simulink model "controller_pid_sim_model_exp_comp"  (R2014b)
settings: Solver=ode45  StartTime=0.0  StopTime=10.0  RelTol=1e-3
values from neighbouring files (symbols this model uses):
  Dr_phi = 0.12*100    (= 12)    [defineGains.m]    (also in gain_tuning.m; model_exp_comparison.m)
  Dr_theta = 0.12*100    (= 12)    [defineGains.m]    (also in gain_tuning.m; model_exp_comparison.m)
  Dvx = 0    [defineGains.m]    (also in gain_tuning.m; model_exp_comparison.m)
  Dvy = 0    [defineGains.m]    (also in gain_tuning.m; model_exp_comparison.m)
  Dx = 0    [defineGains.m]    (also in gain_tuning.m; model_exp_comparison.m)
  Dy = 0    [defineGains.m]    (also in gain_tuning.m; model_exp_comparison.m)
  g = 9.81    [gain_tuning.m]    (also in gain_tuning_noise.m; model_exp_comparison.m; transfer_functions.m)
  Ir_phi = -0.005*100    (= -0.5)    [defineGains.m]    (also in gain_tuning.m; model_exp_comparison.m)
  Ir_theta = -0.005*100    (= -0.5)    [defineGains.m]    (also in gain_tuning.m; model_exp_comparison.m)
  Ivx = -0.05    [defineGains.m]    (also in gain_tuning.m; model_exp_comparison.m)
  Ivy = 0.05    [defineGains.m]    (also in gain_tuning.m; model_exp_comparison.m)
  Ix = 0    [defineGains.m]    (also in gain_tuning.m; model_exp_comparison.m = 0.02)
  Iy = 0    [defineGains.m]    (also in gain_tuning.m; model_exp_comparison.m = 0.03)
  Pa_phi = 10    [defineGains.m]    (also in gain_tuning.m; model_exp_comparison.m)
  Pa_theta = 10    [defineGains.m]    (also in gain_tuning.m; model_exp_comparison.m)
  Pr_phi = 0.2*100    (= 20)    [defineGains.m]    (also in gain_tuning.m; model_exp_comparison.m)
  Pr_theta = 0.2*100    (= 20)    [defineGains.m]    (also in gain_tuning.m; model_exp_comparison.m)
  Pvx = -0.26    [defineGains.m]    (also in gain_tuning.m = -0.35; model_exp_comparison.m)
  Pvy = 0.14    [defineGains.m]    (also in gain_tuning.m = 0.35; model_exp_comparison.m)
  Px = 0.7    [defineGains.m]    (also in gain_tuning.m = 1.5; model_exp_comparison.m = 0.5)
  Py = 0.7    [defineGains.m]    (also in gain_tuning.m = 1.5; model_exp_comparison.m = 0.4)
  vx_sat_max = 1    [gain_tuning.m]    (also in gain_tuning_noise.m = 0.5; model_exp_comparison.m = 0.2)
  vx_sat_min = -1    [gain_tuning.m]    (also in gain_tuning_noise.m = -0.5; model_exp_comparison.m = -0.2)
  vy_sat_max = 1    [gain_tuning.m]    (also in gain_tuning_noise.m = 0.5; model_exp_comparison.m = 0.2)
  vy_sat_min = -1    [gain_tuning.m]    (also in gain_tuning_noise.m = -0.5; model_exp_comparison.m = -0.2)
libraries: simulink x6
settings Model: Creator=MARK  LastModifiedBy=MARK

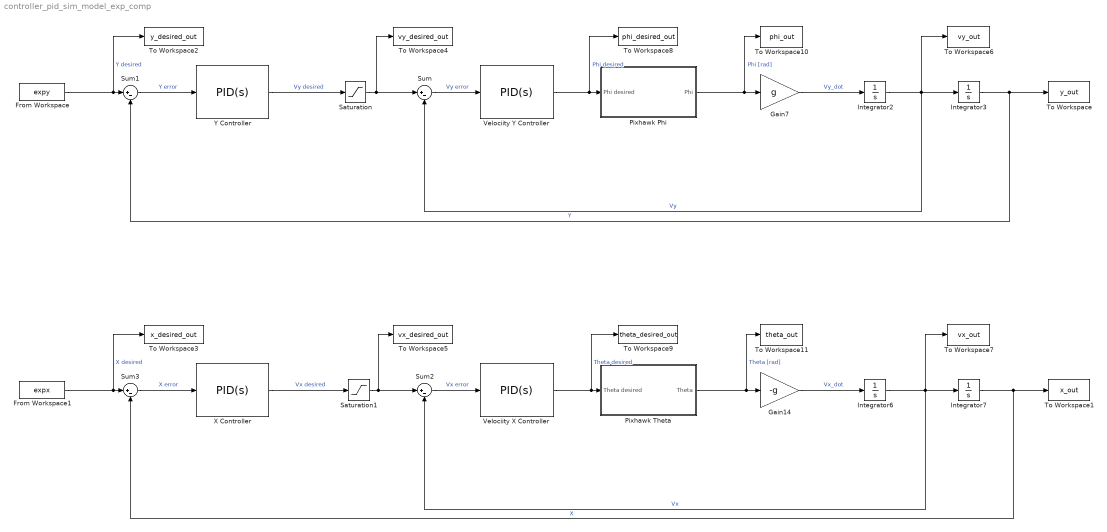
== system controller_pid_sim_model_exp_comp ==
  From Workspace : FromWorkspace  VariableName=expy  SampleTime=0
  From Workspace1 : FromWorkspace  VariableName=expx  SampleTime=0
  Gain14 : Gain  Gain=-g
  Gain7 : Gain  Gain=g
  Integrator{2..3,6..7} (4 alike) : Integrator
  Pixhawk Phi : Subsystem
  Pixhawk Theta : Subsystem
  Saturation : Saturate  UpperLimit=vx_sat_max  LowerLimit=vx_sat_min
  Saturation1 : Saturate  UpperLimit=vy_sat_max  LowerLimit=vy_sat_min
  Sum{,1..3} (4 alike) : Sum  Inputs=|+-
  To Workspace : ToWorkspace  VariableName=y_out  SaveFormat=Structure With Time  SampleTime=-1
  To Workspace1 : ToWorkspace  VariableName=x_out  SaveFormat=Structure With Time  SampleTime=-1
  To Workspace10 : ToWorkspace  VariableName=phi_out  SaveFormat=Structure With Time  SampleTime=-1
  To Workspace11 : ToWorkspace  VariableName=theta_out  SaveFormat=Structure With Time  SampleTime=-1
  To Workspace2 : ToWorkspace  VariableName=y_desired_out  SaveFormat=Structure With Time  SampleTime=-1
  To Workspace3 : ToWorkspace  VariableName=x_desired_out  SaveFormat=Structure With Time  SampleTime=-1
  To Workspace4 : ToWorkspace  VariableName=vy_desired_out  SaveFormat=Structure With Time  SampleTime=-1
  To Workspace5 : ToWorkspace  VariableName=vx_desired_out  SaveFormat=Structure With Time  SampleTime=-1
  To Workspace6 : ToWorkspace  VariableName=vy_out  SaveFormat=Structure With Time  SampleTime=-1
  To Workspace7 : ToWorkspace  VariableName=vx_out  SaveFormat=Structure With Time  SampleTime=-1
  To Workspace8 : ToWorkspace  VariableName=phi_desired_out  SaveFormat=Structure With Time  SampleTime=-1
  To Workspace9 : ToWorkspace  VariableName=theta_desired_out  SaveFormat=Structure With Time  SampleTime=-1
  Velociity X Controller : simulink/Continuous/PID Controller  Controller=PID  TimeDomain=Continuous-time  SampleTime=-1  IntegratorMethod=Forward Euler  FilterMethod=Forward Euler  Form=Parallel  P=Pvx  I=Ivx  D=Dvx  N=100  InitialConditionSource=internal  InitialConditionForIntegrator=0  InitialConditionForFilter=0  ExternalReset=none  LimitOutput=off  UpperSaturationLimit=inf  LowerSaturationLimit=-inf  LinearizeAsGain=on  AntiWindupMode=none  Kb=1  TrackingMode=off  Kt=1  PParamMin=[]  PParamMax=[]  IParamMin=[]  IParamMax=[]  DParamMin=[]  DParamMax=[]  NParamMin=[]  NParamMax=[]  KbParamMin=[]  KbParamMax=[]  KtParamMin=[]  KtParamMax=[]  POutMin=[]  POutMax=[]  IOutMin=[]  IOutMax=[]  DOutMin=[]  DOutMax=[]  NOutMin=[]  NOutMax=[]  KbOutMin=[]  KbOutMax=[]  KtOutMin=[]  KtOutMax=[]  IntegratorOutMin=[]  IntegratorOutMax=[]  FilterOutMin=[]  FilterOutMax=[]  SumOutMin=[]  SumOutMax=[]  SumI1OutMin=[]  SumI1OutMax=[]  SumI2OutMin=[]  SumI2OutMax=[]  SumI3OutMin=[]  SumI3OutMax=[]  SumDOutMin=[]  SumDOutMax=[]  SaturationOutMin=[]  SaturationOutMax=[]  IntegratorContinuousStateAttributes=''  IntegratorStateMustResolveToSignalObject=off  IntegratorRTWStateStorageClass=Auto  FilterContinuousStateAttributes=''  FilterStateMustResolveToSignalObject=off  FilterRTWStateStorageClass=Auto  DifferentiatorICPrevScaledInput=0  DifferentiatorOutMin=[]  DifferentiatorOutMax=[]  UseFilter=on
  Velociity Y Controller : simulink/Continuous/PID Controller  Controller=PID  TimeDomain=Continuous-time  SampleTime=-1  IntegratorMethod=Forward Euler  FilterMethod=Forward Euler  Form=Parallel  P=Pvy  I=Ivy  D=Dvy  N=100  InitialConditionSource=internal  InitialConditionForIntegrator=0  InitialConditionForFilter=0  ExternalReset=none  LimitOutput=off  UpperSaturationLimit=inf  LowerSaturationLimit=-inf  LinearizeAsGain=on  AntiWindupMode=none  Kb=1  TrackingMode=off  Kt=1  PParamMin=[]  PParamMax=[]  IParamMin=[]  IParamMax=[]  DParamMin=[]  DParamMax=[]  NParamMin=[]  NParamMax=[]  KbParamMin=[]  KbParamMax=[]  KtParamMin=[]  KtParamMax=[]  POutMin=[]  POutMax=[]  IOutMin=[]  IOutMax=[]  DOutMin=[]  DOutMax=[]  NOutMin=[]  NOutMax=[]  KbOutMin=[]  KbOutMax=[]  KtOutMin=[]  KtOutMax=[]  IntegratorOutMin=[]  IntegratorOutMax=[]  FilterOutMin=[]  FilterOutMax=[]  SumOutMin=[]  SumOutMax=[]  SumI1OutMin=[]  SumI1OutMax=[]  SumI2OutMin=[]  SumI2OutMax=[]  SumI3OutMin=[]  SumI3OutMax=[]  SumDOutMin=[]  SumDOutMax=[]  SaturationOutMin=[]  SaturationOutMax=[]  IntegratorContinuousStateAttributes=''  IntegratorStateMustResolveToSignalObject=off  IntegratorRTWStateStorageClass=Auto  FilterContinuousStateAttributes=''  FilterStateMustResolveToSignalObject=off  FilterRTWStateStorageClass=Auto  DifferentiatorICPrevScaledInput=0  DifferentiatorOutMin=[]  DifferentiatorOutMax=[]  UseFilter=on
  X Controller : simulink/Continuous/PID Controller  Controller=PID  TimeDomain=Continuous-time  SampleTime=-1  IntegratorMethod=Forward Euler  FilterMethod=Forward Euler  Form=Parallel  P=Px  I=Ix  D=Dx  N=100  InitialConditionSource=internal  InitialConditionForIntegrator=0  InitialConditionForFilter=0  ExternalReset=none  LimitOutput=off  UpperSaturationLimit=inf  LowerSaturationLimit=-inf  LinearizeAsGain=on  AntiWindupMode=none  Kb=1  TrackingMode=off  Kt=1  PParamMin=[]  PParamMax=[]  IParamMin=[]  IParamMax=[]  DParamMin=[]  DParamMax=[]  NParamMin=[]  NParamMax=[]  KbParamMin=[]  KbParamMax=[]  KtParamMin=[]  KtParamMax=[]  POutMin=[]  POutMax=[]  IOutMin=[]  IOutMax=[]  DOutMin=[]  DOutMax=[]  NOutMin=[]  NOutMax=[]  KbOutMin=[]  KbOutMax=[]  KtOutMin=[]  KtOutMax=[]  IntegratorOutMin=[]  IntegratorOutMax=[]  FilterOutMin=[]  FilterOutMax=[]  SumOutMin=[]  SumOutMax=[]  SumI1OutMin=[]  SumI1OutMax=[]  SumI2OutMin=[]  SumI2OutMax=[]  SumI3OutMin=[]  SumI3OutMax=[]  SumDOutMin=[]  SumDOutMax=[]  SaturationOutMin=[]  SaturationOutMax=[]  IntegratorContinuousStateAttributes=''  IntegratorStateMustResolveToSignalObject=off  IntegratorRTWStateStorageClass=Auto  FilterContinuousStateAttributes=''  FilterStateMustResolveToSignalObject=off  FilterRTWStateStorageClass=Auto  DifferentiatorICPrevScaledInput=0  DifferentiatorOutMin=[]  DifferentiatorOutMax=[]  UseFilter=on
  Y Controller : simulink/Continuous/PID Controller  Controller=PID  TimeDomain=Continuous-time  SampleTime=-1  IntegratorMethod=Forward Euler  FilterMethod=Forward Euler  Form=Parallel  P=Py  I=Iy  D=Dy  N=100  InitialConditionSource=internal  InitialConditionForIntegrator=0  InitialConditionForFilter=0  ExternalReset=none  LimitOutput=off  UpperSaturationLimit=inf  LowerSaturationLimit=-inf  LinearizeAsGain=on  AntiWindupMode=none  Kb=1  TrackingMode=off  Kt=1  PParamMin=[]  PParamMax=[]  IParamMin=[]  IParamMax=[]  DParamMin=[]  DParamMax=[]  NParamMin=[]  NParamMax=[]  KbParamMin=[]  KbParamMax=[]  KtParamMin=[]  KtParamMax=[]  POutMin=[]  POutMax=[]  IOutMin=[]  IOutMax=[]  DOutMin=[]  DOutMax=[]  NOutMin=[]  NOutMax=[]  KbOutMin=[]  KbOutMax=[]  KtOutMin=[]  KtOutMax=[]  IntegratorOutMin=[]  IntegratorOutMax=[]  FilterOutMin=[]  FilterOutMax=[]  SumOutMin=[]  SumOutMax=[]  SumI1OutMin=[]  SumI1OutMax=[]  SumI2OutMin=[]  SumI2OutMax=[]  SumI3OutMin=[]  SumI3OutMax=[]  SumDOutMin=[]  SumDOutMax=[]  SaturationOutMin=[]  SaturationOutMax=[]  IntegratorContinuousStateAttributes=''  IntegratorStateMustResolveToSignalObject=off  IntegratorRTWStateStorageClass=Auto  FilterContinuousStateAttributes=''  FilterStateMustResolveToSignalObject=off  FilterRTWStateStorageClass=Auto  DifferentiatorICPrevScaledInput=0  DifferentiatorOutMin=[]  DifferentiatorOutMax=[]  UseFilter=on
  wires:
  Pixhawk Phi/1(Phi) -> To Workspace10/1, Gain7/1  "Phi [rad]"
  Gain7/1 -> Integrator2/1  "Vy_dot"
  Integrator2/1 -> To Workspace6/1, Sum/2, Integrator3/1  "Vy"
  Integrator3/1 -> Sum1/2, To Workspace/1  "Y"
  From Workspace/1 -> To Workspace2/1, Sum1/1  "Y desired"
  Gain14/1 -> Integrator6/1  "Vx_dot"
  Integrator6/1 -> To Workspace7/1, Sum2/2, Integrator7/1  "Vx"
  Integrator7/1 -> Sum3/2, To Workspace1/1  "X"
  From Workspace1/1 -> To Workspace3/1, Sum3/1  "X desired"
  Pixhawk Theta/1(Theta) -> To Workspace11/1, Gain14/1  "Theta [rad]"
  Velociity Y Controller/1 -> To Workspace8/1, Pixhawk Phi/1(Phi desired)  "Phi desired"
  Sum/1 -> Velociity Y Controller/1  "Vy error"
  Y Controller/1 -> Saturation/1  "Vy desired"
  Sum1/1 -> Y Controller/1  "Y error"
  Velociity X Controller/1 -> To Workspace9/1, Pixhawk Theta/1(Theta desired)  "Theta desired"
  Sum2/1 -> Velociity X Controller/1  "Vx error"
  X Controller/1 -> Saturation1/1  "Vx desired"
  Sum3/1 -> X Controller/1  "X error"
  Saturation/1 -> To Workspace4/1, Sum/1
  Saturation1/1 -> To Workspace5/1, Sum2/1

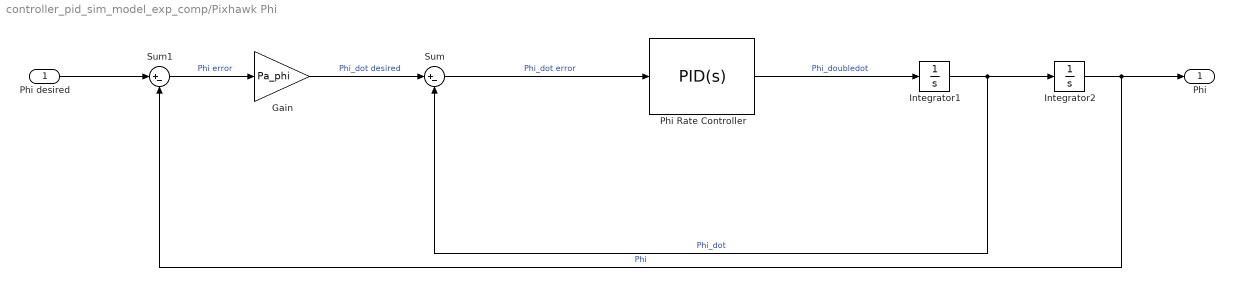
== system controller_pid_sim_model_exp_comp/Pixhawk Phi ==
  Phi desired : Inport
  Gain : Gain  Gain=Pa_phi
  Integrator1 : Integrator
  Integrator2 : Integrator
  Phi Rate Controller : simulink/Continuous/PID Controller  Controller=PID  TimeDomain=Continuous-time  SampleTime=-1  IntegratorMethod=Forward Euler  FilterMethod=Forward Euler  Form=Parallel  P=Pr_phi  I=Ir_phi  D=Dr_phi  N=100  InitialConditionSource=internal  InitialConditionForIntegrator=0  InitialConditionForFilter=0  ExternalReset=none  LimitOutput=off  UpperSaturationLimit=inf  LowerSaturationLimit=-inf  LinearizeAsGain=on  AntiWindupMode=none  Kb=1  TrackingMode=off  Kt=1  PParamMin=[]  PParamMax=[]  IParamMin=[]  IParamMax=[]  DParamMin=[]  DParamMax=[]  NParamMin=[]  NParamMax=[]  KbParamMin=[]  KbParamMax=[]  KtParamMin=[]  KtParamMax=[]  POutMin=[]  POutMax=[]  IOutMin=[]  IOutMax=[]  DOutMin=[]  DOutMax=[]  NOutMin=[]  NOutMax=[]  KbOutMin=[]  KbOutMax=[]  KtOutMin=[]  KtOutMax=[]  IntegratorOutMin=[]  IntegratorOutMax=[]  FilterOutMin=[]  FilterOutMax=[]  SumOutMin=[]  SumOutMax=[]  SumI1OutMin=[]  SumI1OutMax=[]  SumI2OutMin=[]  SumI2OutMax=[]  SumI3OutMin=[]  SumI3OutMax=[]  SumDOutMin=[]  SumDOutMax=[]  SaturationOutMin=[]  SaturationOutMax=[]  IntegratorContinuousStateAttributes=''  IntegratorStateMustResolveToSignalObject=off  IntegratorRTWStateStorageClass=Auto  FilterContinuousStateAttributes=''  FilterStateMustResolveToSignalObject=off  FilterRTWStateStorageClass=Auto  DifferentiatorICPrevScaledInput=0  DifferentiatorOutMin=[]  DifferentiatorOutMax=[]  UseFilter=on
  Sum : Sum  Inputs=|+-
  Sum1 : Sum  Inputs=|+-
  Phi : Outport
  wires:
  Integrator2/1 -> Phi/1, Sum1/2  "Phi"
  Integrator1/1 -> Sum/2, Integrator2/1  "Phi_dot"
  Gain/1 -> Sum/1  "Phi_dot desired"
  Phi desired/1 -> Sum1/1
  Sum1/1 -> Gain/1  "Phi error"
  Phi Rate Controller/1 -> Integrator1/1  "Phi_doubledot"
  Sum/1 -> Phi Rate Controller/1  "Phi_dot error"

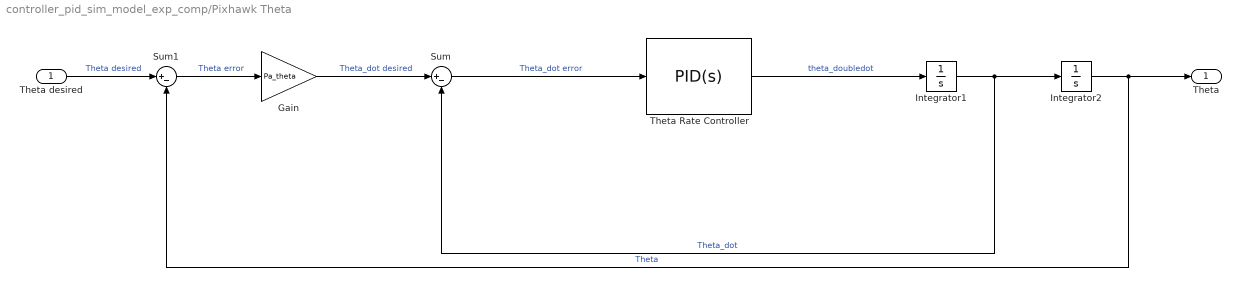
== system controller_pid_sim_model_exp_comp/Pixhawk Theta ==
  Theta desired : Inport
  Gain : Gain  Gain=Pa_theta
  Integrator1 : Integrator
  Integrator2 : Integrator
  Sum : Sum  Inputs=|+-
  Sum1 : Sum  Inputs=|+-
  Theta Rate Controller : simulink/Continuous/PID Controller  Controller=PID  TimeDomain=Continuous-time  SampleTime=-1  IntegratorMethod=Forward Euler  FilterMethod=Forward Euler  Form=Parallel  P=Pr_theta  I=Ir_theta  D=Dr_theta  N=100  InitialConditionSource=internal  InitialConditionForIntegrator=0  InitialConditionForFilter=0  ExternalReset=none  LimitOutput=off  UpperSaturationLimit=inf  LowerSaturationLimit=-inf  LinearizeAsGain=on  AntiWindupMode=none  Kb=1  TrackingMode=off  Kt=1  PParamMin=[]  PParamMax=[]  IParamMin=[]  IParamMax=[]  DParamMin=[]  DParamMax=[]  NParamMin=[]  NParamMax=[]  KbParamMin=[]  KbParamMax=[]  KtParamMin=[]  KtParamMax=[]  POutMin=[]  POutMax=[]  IOutMin=[]  IOutMax=[]  DOutMin=[]  DOutMax=[]  NOutMin=[]  NOutMax=[]  KbOutMin=[]  KbOutMax=[]  KtOutMin=[]  KtOutMax=[]  IntegratorOutMin=[]  IntegratorOutMax=[]  FilterOutMin=[]  FilterOutMax=[]  SumOutMin=[]  SumOutMax=[]  SumI1OutMin=[]  SumI1OutMax=[]  SumI2OutMin=[]  SumI2OutMax=[]  SumI3OutMin=[]  SumI3OutMax=[]  SumDOutMin=[]  SumDOutMax=[]  SaturationOutMin=[]  SaturationOutMax=[]  IntegratorContinuousStateAttributes=''  IntegratorStateMustResolveToSignalObject=off  IntegratorRTWStateStorageClass=Auto  FilterContinuousStateAttributes=''  FilterStateMustResolveToSignalObject=off  FilterRTWStateStorageClass=Auto  DifferentiatorICPrevScaledInput=0  DifferentiatorOutMin=[]  DifferentiatorOutMax=[]  UseFilter=on
  Theta : Outport
  wires:
  Integrator2/1 -> Theta/1, Sum1/2  "Theta"
  Integrator1/1 -> Sum/2, Integrator2/1  "Theta_dot"
  Gain/1 -> Sum/1  "Theta_dot desired"
  Theta desired/1 -> Sum1/1  "Theta desired"
  Sum1/1 -> Gain/1  "Theta error"
  Theta Rate Controller/1 -> Integrator1/1  "theta_doubledot"
  Sum/1 -> Theta Rate Controller/1  "Theta_dot error"
